simulink model "Brk_DD"  (R2016b)
settings: configuration reference "CodeGenConfigSet" (kept outside this file)
values from neighbouring files (symbols this model uses):
  Brk_tiMnDebHiLo_C = Calibration.Parameter    [init_Brk_DD.m]
  Brk_tiMnDebLoHi_C = Calibration.Parameter    [init_Brk_DD.m]
  Brk_tiRedDebHiLo_C = Calibration.Parameter    [init_Brk_DD.m]
  Brk_tiRedDebLoHi_C = Calibration.Parameter    [init_Brk_DD.m]
  BrkDD_bBrkSigInv_C = Calibration.Parameter    [init_Brk_DD.m]
  SigTst_stBrkMn_C = Calibration.Parameter    [init_Brk_DD.m]
  SigTst_stBrkRed_C = Calibration.Parameter    [init_Brk_DD.m]
  SigTst_swtBrkMn_C = Calibration.Parameter    [init_Brk_DD.m]
  SigTst_swtBrkRed_C = Calibration.Parameter    [init_Brk_DD.m]
undefined symbols (not defined in the file or in its folder): Brk_DD_DT, Switch_conv
libraries: CXLib x2
settings Model: Creator=lenovo  LastModifiedBy=bianxuyin
settings ConfigSetRef: SourceLocation=Base Workspace

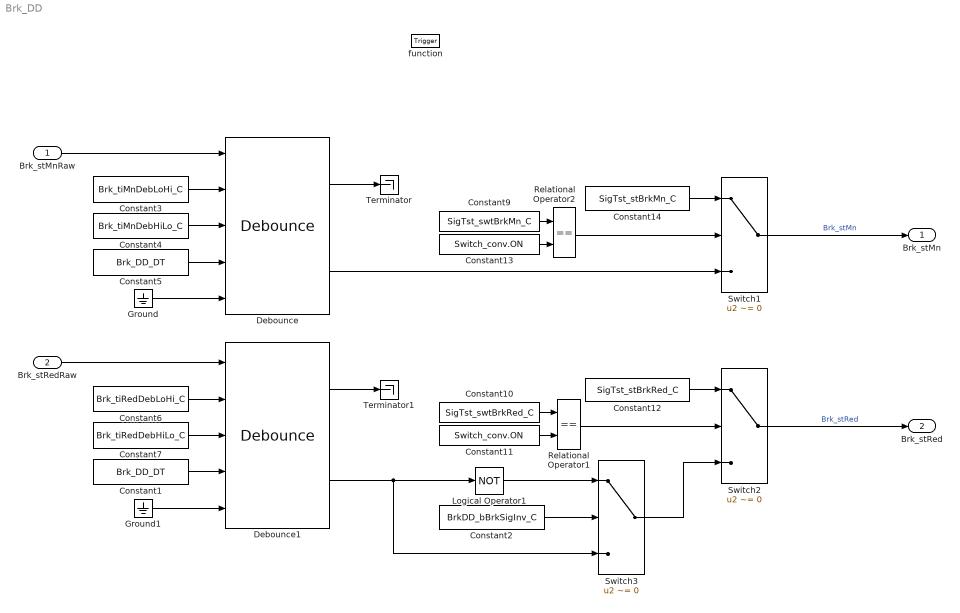
== system Brk_DD ==
  Brk_stMnRaw : Inport  Description=State main brake switch, raw value  OutMin=0  OutMax=1  OutDataTypeStr=boolean
  Brk_stRedRaw : Inport  Description=State redundant brake switch, raw value  Port=2  OutMin=0  OutMax=1  OutDataTypeStr=boolean
  function : TriggerPort  TriggerType=function-call  VariantControl=Variant
  Constant1 : Constant  Value=Brk_DD_DT  OutDataTypeStr=Inherit: Inherit via back propagation
  Constant10 : Constant  Value=SigTst_swtBrkRed_C
  Constant11 : Constant  Value=Switch_conv.ON
  Constant12 : Constant  Value=SigTst_stBrkRed_C
  Constant13 : Constant  Value=Switch_conv.ON
  Constant14 : Constant  Value=SigTst_stBrkMn_C
  Constant2 : Constant  Value=BrkDD_bBrkSigInv_C
  Constant3 : Constant  Value=Brk_tiMnDebLoHi_C
  Constant4 : Constant  Value=Brk_tiMnDebHiLo_C
  Constant5 : Constant  Value=Brk_DD_DT  OutDataTypeStr=Inherit: Inherit via back propagation
  Constant6 : Constant  Value=Brk_tiRedDebLoHi_C
  Constant7 : Constant  Value=Brk_tiRedDebHiLo_C
  Constant9 : Constant  Value=SigTst_swtBrkMn_C
  Debounce : CXLib/Debounce
  Debounce1 : CXLib/Debounce
  Ground : Ground
  Ground1 : Ground
  Logical Operator1 : Logic  Operator=NOT  OutDataTypeStr=boolean
  Relational Operator1 : RelationalOperator  Operator===  OutDataTypeStr=boolean  RndMeth=Nearest
  Relational Operator2 : RelationalOperator  Operator===  OutDataTypeStr=boolean  RndMeth=Nearest
  Switch1 : Switch  Criteria=u2 ~= 0  OutDataTypeStr=Inherit: Inherit via back propagation  SaturateOnIntegerOverflow=on  InputSameDT=on
  Switch2 : Switch  Criteria=u2 ~= 0  OutDataTypeStr=Inherit: Inherit via back propagation  SaturateOnIntegerOverflow=on  InputSameDT=on
  Switch3 : Switch  Criteria=u2 ~= 0  OutDataTypeStr=Inherit: Inherit via back propagation  SaturateOnIntegerOverflow=on  InputSameDT=on
  Terminator : Terminator
  Terminator1 : Terminator
  Brk_stMn : Outport  Description=Status of the main brake  OutMin=0  OutMax=1  OutDataTypeStr=boolean
  Brk_stRed : Outport  Description=Status of the redundant break  Port=2  OutMin=0  OutMax=1  OutDataTypeStr=boolean
  wires:
  Switch2/1 -> Brk_stRed/1  "Brk_stRed"
  Constant12/1 -> Switch2/1
  Relational Operator1/1 -> Switch2/2
  Constant10/1 -> Relational Operator1/1
  Constant11/1 -> Relational Operator1/2
  Switch1/1 -> Brk_stMn/1  "Brk_stMn"
  Constant14/1 -> Switch1/1
  Relational Operator2/1 -> Switch1/2
  Constant9/1 -> Relational Operator2/1
  Constant13/1 -> Relational Operator2/2
  Debounce1/1 -> Terminator1/1
  Debounce/1 -> Terminator/1
  Debounce/2 -> Switch1/3
  Brk_stRedRaw/1 -> Debounce1/1
  Ground1/1 -> Debounce1/5
  Constant1/1 -> Debounce1/4
  Constant7/1 -> Debounce1/3
  Constant6/1 -> Debounce1/2
  Ground/1 -> Debounce/5
  Constant5/1 -> Debounce/4
  Constant4/1 -> Debounce/3
  Constant3/1 -> Debounce/2
  Brk_stMnRaw/1 -> Debounce/1
  Logical Operator1/1 -> Switch3/1
  Debounce1/2 -> Switch3/3, Logical Operator1/1
  Constant2/1 -> Switch3/2
  Switch3/1 -> Switch2/3
